simulink model "mfcm_cosim"  (Simulink 7.1)
settings: Solver=VariableStepDiscrete  StartTime=0.0  StopTime=256  RelTol=1e-3
undefined symbols (not defined in the file): mimo_setup
libraries: xbsIndex_r4 x3, xbsCopyrightNotice_r4 x1, JTAGRuntimeCosim_r4 x1
settings Model: Creator=alexc  LastModifiedBy=bchan
settings OptimizationCC: InlineInvariantSignals=on
settings DebuggingCC: SaveWithParameterizedLinksMsg=none  SignalResolutionControl=TryResolveAllWithWarning  SolverPrmCheckMsg=none  MultiTaskDSMMsg=warning  MultiTaskCondExecSysMsg=none  StrictBusMsg=None
settings RTWCC: IncludeERTFirstTime=on
settings GRTTargetCC: TargetFcnLib=ansi_tfl_tmw.mat

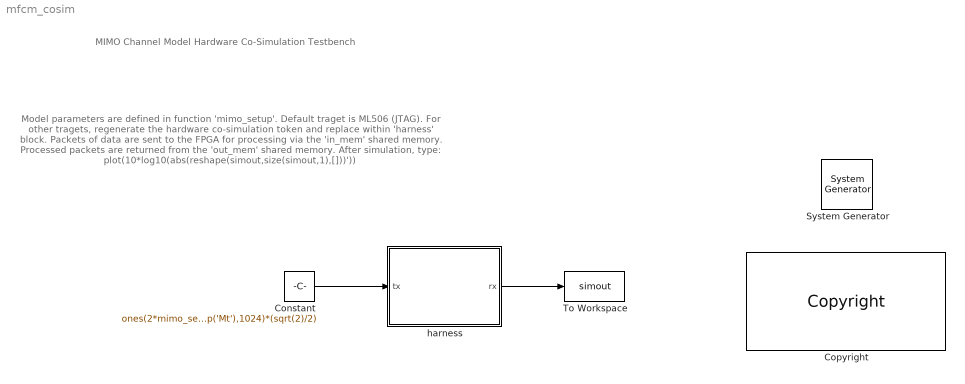
== system mfcm_cosim ==
  note: Model parameters are defined in function 'mimo_setup'.
      |
      | Default traget is ML506 (JTAG).
      | For other tragets, regenerate the hardware co-simulation token and replace within 'harness' block.
      |
      | Packets of data are sent to the FPGA for processing via the 'in_mem' shared memory.
      | Processed packets are returned from the 'out_mem' shared memory.
      |
      | After simulation, type:
      |     plot(10*log10(abs(reshape(simout,size(simout,1),[]))'))
  note: MIMO Channel Model Hardware Co-Simulation Testbench
  " System Generator" : xbsIndex_r4/ System Generator  Tag=genX  SystemSampleTime=-1  xilinxfamily=Virtex2  part=xc2v3000  speed=-4  package=fg676  synthesis_tool=XST  clock_wrapper=Clock Enables  directory=./netlist  testbench=off  simulink_period=1  sysclk_period=20  dcm_input_clock_period=10  incr_netlist=off  trim_vbits=Everywhere in SubSystem  dbl_ovrd=According to Block Masks  core_generation=According to Block Masks  run_coregen=off  deprecated_control=off  eval_field=0  block_type=sysgen
      settings: block_version=11.3
  Constant : Constant  Value=ones(2*mimo_setup('Mt'),1024)*(sqrt(2)/2)  OutDataTypeMode=double  OutDataType=sfix(16)  OutScaling=2^0  OutDataTypeStr=double
  Copyright : xbsCopyrightNotice_r4/Copyright  copyrighttext="Copyright (c) 2009  by  Xilinx, Inc. All rights reserved.<br><br>This file contains proprietary, confidential information of Xilinx, Inc., is distributed under licensefrom Xilinx, Inc., and may be used, copied and/or disclosed only pursuant to the terms of a valid licenseagreement with Xilinx, Inc. Xilinx hereby grants you a license to use this file solely for design,simulation, implementation and creation of design files limited to Xilinx devices or technologies. Use with non-Xilinx devices or technologies is expressly prohibited and immediately terminates your license unless covered by a separate agreement.<br><br>Xilinx is providing this design, code, or information \"as-is\" solely for use in developing programs and solutions for Xilinx devices, with no obligation on the part of Xilinx to provide support. By providingthis design, code, or information as one possible implementation of this feature, application or standard,Xilinx is making no representation that this implementation is free from any claims of infringement. Youare responsible for obtaining any rights you may require for your implementation. Xilinx expressly disclaimsany warranty whatsoever with respect to the adequacy of the implementation, including but not limited to anywarranties or representations that this implementation is free from claims of infringement, implied warrantiesof merchantability or fitness for a particular purpose.<br><br>Xilinx products are not intended for use in life support appliances, devices, or systems. Use in such applications is expressly prohibited.<br><br>Any modifications that are made to the Source Code are done at the user's sole risk and will be unsupported.<br><br>This copyright and support notice must be retained as part of this text at all times. (c) Copyright 1995-2009 Xilinx, Inc. All rights reserved."  block_type=copyright
      settings: block_version=11.3
  To Workspace : ToWorkspace  VariableName=simout  SampleTime=-1  SaveFormat=Array
  harness : Subsystem  mask{MT=mimo_setup('Mt'), MR=mimo_setup('Mr'), LEN=1024}
      mask prompts: MT "Number of Tx Antennas"; MR "Number of Rx Antennas"; LEN "Burst Length"
  wires:
  Constant/1 -> harness/1(tx)
  harness/1(rx) -> To Workspace/1

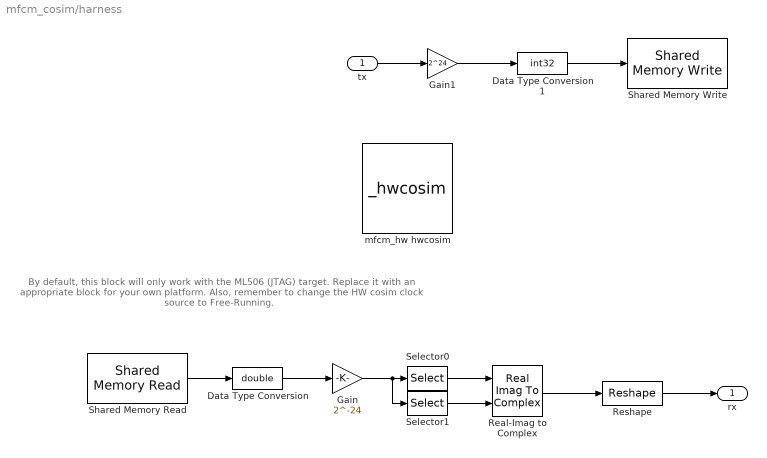
== system mfcm_cosim/harness ==
  note: By default, this block will only work with the ML506 (JTAG) target.
      | Replace it with an appropriate block for your own platform.
      | Also, remember to change the HW cosim clock source to Free-Running.
  tx : Inport  OutDataType=sfix(16)  OutScaling=2^0
  Data Type Conversion : DataTypeConversion  OutDataTypeMode=double  OutDataType=sfix(16)  OutScaling=2^0  OutDataTypeStr=double
  Data Type Conversion1 : DataTypeConversion  OutDataTypeMode=int32  OutDataType=sfix(16)  OutScaling=2^0  OutDataTypeStr=int32
  Gain : Gain  Gain=2^-24  ParameterDataType=sfix(16)  ParameterScaling=2^0  OutDataType=sfix(16)  OutScaling=2^0
  Gain1 : Gain  Gain=2^24  ParameterDataType=sfix(16)  ParameterScaling=2^0  OutDataType=sfix(16)  OutScaling=2^0
  Real-Imag to Complex : RealImagToComplex
  Reshape : Reshape  OutputDimensionality=Customize  OutputDimensions=[MR LEN]
  Selector0 : Selector  NumberOfDimensions=2  InputPortWidth=3  IndexOptions=Index vector (dialog),Select all  Indices=1,-1  OutputSizes=1
  Selector1 : Selector  NumberOfDimensions=2  InputPortWidth=3  IndexOptions=Index vector (dialog),Select all  Indices=2,-1  OutputSizes=1
  Shared Memory Read : xbsIndex_r4/Shared Memory Read  Priority=10  shmem_name='out_mem'  shmem_type=Lockable memory  sample_time=1  dataType=int32  outDims=[2 MR*LEN]  isFrame=off  shmem_word=32  shmem_depth=8192  block_type=fromshmem
      settings: AttributesFormatString=<< %<shmem_name> >>  infoedit=Reads sequentially from a shared memory block.  block_version=VER_STRING_GOES_HERE
  Shared Memory Write : xbsIndex_r4/Shared Memory Write  Priority=-10  shmem_name='in_mem'  shmem_type=Lockable memory  skip_check=0  shmem_word=32  shmem_depth=8192  block_type=toshmem
      settings: AttributesFormatString=<< %<shmem_name> >>  infoedit=Writes scalar, vector, matrix, or frame data into a shared memory.  block_version=VER_STRING_GOES_HERE
  mfcm_hw hwcosim : JTAGRuntimeCosim_r4/_hwcosim  clkSrc=Free Running  hasCombinationalPath=on  bitfileName=.\mfcm_hw_cw.bit  skipConfig=off  cable=Xilinx Platform USB  speed=12 MHz  shareCable=off  treeview=|  design_xtable=|  engineDll=JTAGCosimEngine.dll  bscanPos=5  IRLengths=[16,16,8,8,10]  useWaitBox=1  hasBufgmux=on  Scheme=Cosim  useCmdProc=1  memxtable={'treeview'=>[{'icon'=>'memory','label'=>'&lt;&lt;&apos;in_mem&apos;&gt;&gt;','param'=>['Depth: 8192','Number of Bits: 32','Access Protection: Lockable'],'state'=>0.00000000000000000},{'icon'=>'memory','label'=>'&lt;&lt;&apos;out_mem&apos;&gt;&gt;','param'=>['Depth: 8192','Number of Bits: 32','Access Protection: Lockable'],'state'=>0.00000000000000000}]}  hasProc=0  block_type=jtagcosim
      treeview=|
      | <!DOCTYPE HTML PUBLIC "-//W3C//DTD HTML 4.0//EN" "http://www.w3.org/TR/REC-html40/strict.dtd">
      | <html><head><meta name="qrichtext" content="1" /><style type="text/css">
      | p, li { white-space: pre-wrap; }
      | </style></head><body style=" font-family:'MS Shell Dlg 2'; font-size:8.25pt; font-weight:400; font-style:normal;" bgcolor="#ffffff">
      | <p style=" margin-top:0px; margin-bottom:0px; margin-left:0px; margin-right:0px; -qt-block-indent:0; text-indent:0px;"><img src="D:/repos/svn/sg/trunk/output/debug/export/sysgen/data/images//memoryplus.gif" /> &lt;&lt;'in_mem'&gt;&gt;</p>
      | <p style=" margin-top:0px; margin-bottom:0px; margin-left:0px; margin-right:0px; -qt-block-indent:0; text-indent:0px;"><img src="D:/repos/svn/sg/trunk/output/debug/export/sysgen/data/images//memoryplus.gif" /> &lt;&lt;'out_mem'&gt;&gt;</p></body></html>
      design_xtable=|
      | {
      |   'clkWrapper' => 'mfcm_hw_cw',
      |   'clocksGcd' => undef,
      |   'device' => 'xc5vsx50t-1ff1136',
      |   'ports' => {},
      |   'shared_memories' => {
      |     'in_mem' => {
      |       'bank' => 1,
      |       'block_config' => 'sysgen_blockset:shmem_config',
      |       'depth' => 8192,
      |       'grant_index' => 0,
      |       'mutex' => 0,
      |       'request_index' => 0,
      |       'width' => 32,
      |       'write_mode' => 3,
      |     },
      |     'out_mem' => {
      |       'bank' => 2,
      |       'block_config' => 'sysgen_blockset:shmem_config',
      |       'depth' => 8192,
      |       'grant_index' => 1,
      |       'mutex' => 0,
      |       'request_index' => 1,
      |       'width' => 32,
      |       'write_mode' => 3,
      |     },
      |   },
      | }
      settings: block_version=11.3
  rx : Outport  OutDataType=sfix(16)  OutScaling=2^0
  wires:
  Shared Memory Read/1 -> Data Type Conversion/1
  Data Type Conversion/1 -> Gain/1
  Gain/1 -> Selector0/1, Selector1/1
  Selector0/1 -> Real-Imag to Complex/1
  Selector1/1 -> Real-Imag to Complex/2
  tx/1 -> Gain1/1
  Real-Imag to Complex/1 -> Reshape/1
  Reshape/1 -> rx/1
  Gain1/1 -> Data Type Conversion1/1
  Data Type Conversion1/1 -> Shared Memory Write/1
